simulink model "flightController"  (R2021b)
settings: Solver=ode3  StartTime=0  StopTime=TFinal  FixedStep=Ts  RelTol=1e-3  EnableMultiTasking=on
undefined symbols (not defined in the file): Controller, DiscIntNeverNeededParam, g, INDI, Ts, Vehicle
libraries: spsSecondOrderFilterLib x12, simulink x6
settings Model: Creator=The MathWorks, Inc.  LastModifiedBy=Tiga
settings SolverCC: AlgebraicLoopSolver=TrustRegion  MinimalZcImpactIntegration=on
settings DataIOCC: LimitDataPoints=on  SaveFormat=Array  ReturnWorkspaceOutputs=off
settings OptimizationCC: BlockReduction=off  DefaultParameterBehavior=Inlined  BufferReuse=off  PassReuseOutputArgsThreshold=0
settings DebuggingCC: AlgebraicLoopMsg=none  ParameterPrecisionLossMsg=none  ParameterTunabilityLossMsg=error  UnconnectedInputMsg=none  UnconnectedOutputMsg=none  UnconnectedLineMsg=none  BusObjectLabelMismatch=error  SFUnexpectedBacktrackingDiag=warning  SFNoUnconditionalDefaultTransitionDiag=warning  SFExecutionAtInitializationDiag=none  SFMachineParentedDataDiag=warning  ArithmeticOperatorsInVariantConditions=warning
settings HardwareCC: ProdBitPerPointer=32  ProdBitPerSizeT=32  ProdBitPerPtrDiffT=32  ProdLargestAtomicInteger=Long  ProdWordSize=32  ProdHWDeviceType=ARM Compatible->ARM 9
settings ModelReferenceCC: ModelReferenceNumInstancesAllowed=Single  PropagateSignalLabelsOutOfModel=off
settings SFSimCC: SimUseLocalCustomCode=off  CustomCodeUndefinedFunction=UseInterfaceOnly
settings RTWCC: GenerateReport=on  RTWUseLocalCustomCode=off  LaunchReport=on
settings CodeAppCC: ForceParamTrailComments=on  MaxIdLength=63  OperatorAnnotations=on  StateflowObjectComments=on  MATLABSourceComments=on
settings GRTTargetCC: TargetLangStandard=C89/C90 (ANSI)
settings ConfigComp: CovMetricSettings=dw  CovSaveCumulativeToWorkspaceVar=on  CovSaveSingleToWorkspaceVar=on  CovExternalEMLEnable=off  CovSFcnEnable=off

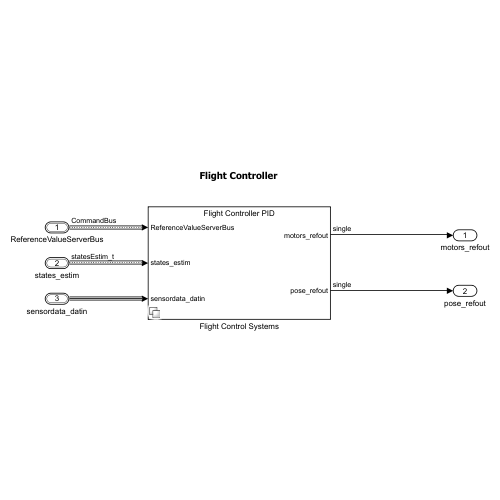
[thumbnail: Simulink's stored preview of the top-level diagram]
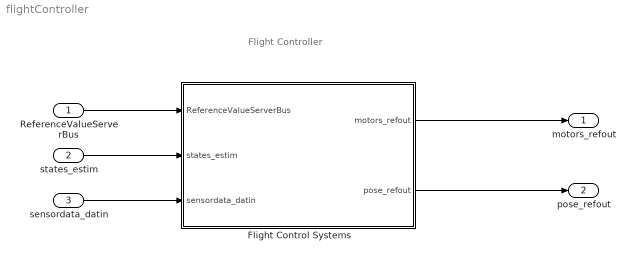
== system flightController ==
  note: Flight Controller
  ReferenceValueServerBus : Inport  OutDataTypeStr=Bus: CommandBus  BusOutputAsStruct=on
  states_estim : Inport  Port=2  OutDataTypeStr=Bus: statesEstim_t  BusOutputAsStruct=on
  sensordata_datin : Inport  Port=3  OutDataTypeStr=Bus: sensordata_t
  Flight Control Systems : Subsystem  Variant=on
  motors_refout : Outport  VectorParamsAs1DForOutWhenUnconnected=off
  pose_refout : Outport  Port=2  VectorParamsAs1DForOutWhenUnconnected=off
  wires:
  ReferenceValueServerBus/1 -> Flight Control Systems/1(ReferenceValueServerBus)
  states_estim/1 -> Flight Control Systems/2(states_estim)
  Flight Control Systems/2(pose_refout) -> pose_refout/1
  Flight Control Systems/1(motors_refout) -> motors_refout/1
  sensordata_datin/1 -> Flight Control Systems/3(sensordata_datin)

== system flightController/Flight Control Systems ==
  note: 1) Add Subsystem or Model blocks as valid variant choices.
      | 2) You cannot connect blocks at this level. At simulation, connectivity is automatically
      | determined, based on the active variant and port name matching.
  ReferenceValueServerBus : Inport
  states_estim : Inport  Port=2
  sensordata_datin : Inport  Port=3
  Flight Controller INDI : Subsystem  VariantControl=VSS_FCS_INDI
  Flight Controller PID : Subsystem  VariantControl=VSS_FCS_PID
  Flight Controller PID + INDI : Subsystem  VariantControl=VSS_FCS_PID_INDI
  motors_refout : Outport
  pose_refout : Outport  Port=2

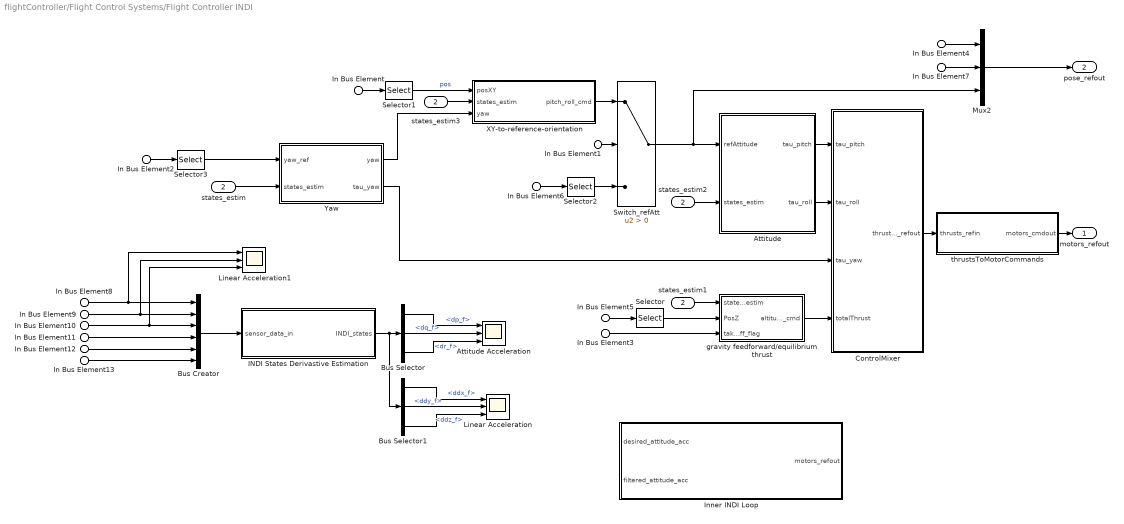
== system flightController/Flight Control Systems/Flight Controller INDI ==
  In Bus Element1 : Inport  PortName=ReferenceValueServerBus  Element=controlModePosVSOrient
  In Bus Element : Inport  PortName=ReferenceValueServerBus  Element=pos_ref
  In Bus Element4 : Inport  PortName=ReferenceValueServerBus  Element=pos_ref
  In Bus Element5 : Inport  PortName=ReferenceValueServerBus  Element=pos_ref
  In Bus Element2 : Inport  PortName=ReferenceValueServerBus  Element=orient_ref
  In Bus Element6 : Inport  PortName=ReferenceValueServerBus  Element=orient_ref
  In Bus Element7 : Inport  PortName=ReferenceValueServerBus  Element=orient_ref
  In Bus Element3 : Inport  PortName=ReferenceValueServerBus  Element=takeoff_flag
  states_estim : Inport  Port=2
  In Bus Element8 : Inport  Port=3  PortName=sensordata_datin  Element=ddx
  In Bus Element9 : Inport  Port=3  PortName=sensordata_datin  Element=ddy
  In Bus Element10 : Inport  Port=3  PortName=sensordata_datin  Element=ddz
  In Bus Element11 : Inport  Port=3  PortName=sensordata_datin  Element=p
  In Bus Element12 : Inport  Port=3  PortName=sensordata_datin  Element=q
  In Bus Element13 : Inport  Port=3  PortName=sensordata_datin  Element=r
  Attitude : Subsystem
  Attitude Acceleration : Scope  NumInputPorts=3
  Bus Creator : BusCreator  Inputs=6
  Bus Selector : BusSelector  OutputSignals=dp_f,dq_f,dr_f
  Bus Selector1 : BusSelector  OutputSignals=ddx_f,ddy_f,ddz_f
  ControlMixer : Subsystem
  INDI States Derivastive Estimation : Subsystem
  Inner INDI Loop : Subsystem
  Linear Acceleration : Scope  NumInputPorts=3
  Linear Acceleration1 : Scope  NumInputPorts=3
  Mux2 : Mux  Inputs=3
  Selector : Selector  InputPortWidth=3  IndexOptions=Index vector (dialog)  Indices=3  OutputSizes=1
  Selector1 : Selector  InputPortWidth=3  IndexOptions=Index vector (dialog)  Indices=[1 2]  OutputSizes=1
  Selector2 : Selector  InputPortWidth=3  IndexOptions=Index vector (dialog)  Indices=[2 3]  OutputSizes=1
  Selector3 : Selector  InputPortWidth=3  IndexOptions=Index vector (dialog)  Indices=1  OutputSizes=1
  Switch_refAtt : Switch  Criteria=u2 > Threshold
  XY-to-reference-orientation : Subsystem
  Yaw : Subsystem
  gravity feedforward/equilibrium thrust : Subsystem
  states_estim1 : InportShadow  Port=2
  states_estim2 : InportShadow  Port=2
  states_estim3 : InportShadow  Port=2
  thrustsToMotorCommands : Subsystem
  motors_refout : Outport  VectorParamsAs1DForOutWhenUnconnected=off
  pose_refout : Outport  Port=2  VectorParamsAs1DForOutWhenUnconnected=off
  wires:
  thrustsToMotorCommands/1(motors_cmdout) -> motors_refout/1
  In Bus Element1/1 -> Switch_refAtt/2
  XY-to-reference-orientation/1(pitch_roll_cmd) -> Switch_refAtt/1
  In Bus Element2/1 -> Selector3/1
  In Bus Element/1 -> Selector1/1
  Selector3/1 -> Yaw/1(yaw_ref)
  Selector1/1 -> XY-to-reference-orientation/1(posXY)  "pos"
  ControlMixer/1(thrusts_refout) -> thrustsToMotorCommands/1(thrusts_refin)
  In Bus Element3/1 -> gravity feedforward/equilibrium thrust/3(takeoff_flag)
  states_estim/1 -> Yaw/2(states_estim)
  Switch_refAtt/1 -> Attitude/1(refAttitude), Mux2/3
  Yaw/1(yaw) -> XY-to-reference-orientation/3(yaw)
  gravity feedforward/equilibrium thrust/1(altitude_cmd) -> ControlMixer/4(totalThrust)
  Mux2/1 -> pose_refout/1
  Attitude/1(tau_pitch) -> ControlMixer/1(tau_pitch)
  Attitude/2(tau_roll) -> ControlMixer/2(tau_roll)
  Yaw/2(tau_yaw) -> ControlMixer/3(tau_yaw)
  states_estim1/1 -> gravity feedforward/equilibrium thrust/1(states_estim)
  states_estim2/1 -> Attitude/2(states_estim)
  states_estim3/1 -> XY-to-reference-orientation/2(states_estim)
  In Bus Element4/1 -> Mux2/1
  Selector/1 -> gravity feedforward/equilibrium thrust/2(PosZ)
  In Bus Element5/1 -> Selector/1
  In Bus Element6/1 -> Selector2/1
  Selector2/1 -> Switch_refAtt/3
  In Bus Element7/1 -> Mux2/2
  INDI States Derivastive Estimation/1(INDI_states) -> Bus Selector1/1, Bus Selector/1
  Bus Selector/1 -> Attitude Acceleration/1  "<dp_f>"
  Bus Selector/2 -> Attitude Acceleration/2  "<dq_f>"
  Bus Selector/3 -> Attitude Acceleration/3  "<dr_f>"
  In Bus Element8/1 -> Bus Creator/1, Linear Acceleration1/1
  In Bus Element9/1 -> Bus Creator/2, Linear Acceleration1/2
  In Bus Element10/1 -> Bus Creator/3, Linear Acceleration1/3
  In Bus Element11/1 -> Bus Creator/4
  In Bus Element13/1 -> Bus Creator/6
  In Bus Element12/1 -> Bus Creator/5
  Bus Creator/1 -> INDI States Derivastive Estimation/1(sensor_data_in)
  Bus Selector1/1 -> Linear Acceleration/1  "<ddx_f>"
  Bus Selector1/2 -> Linear Acceleration/2  "<ddy_f>"
  Bus Selector1/3 -> Linear Acceleration/3  "<ddz_f>"

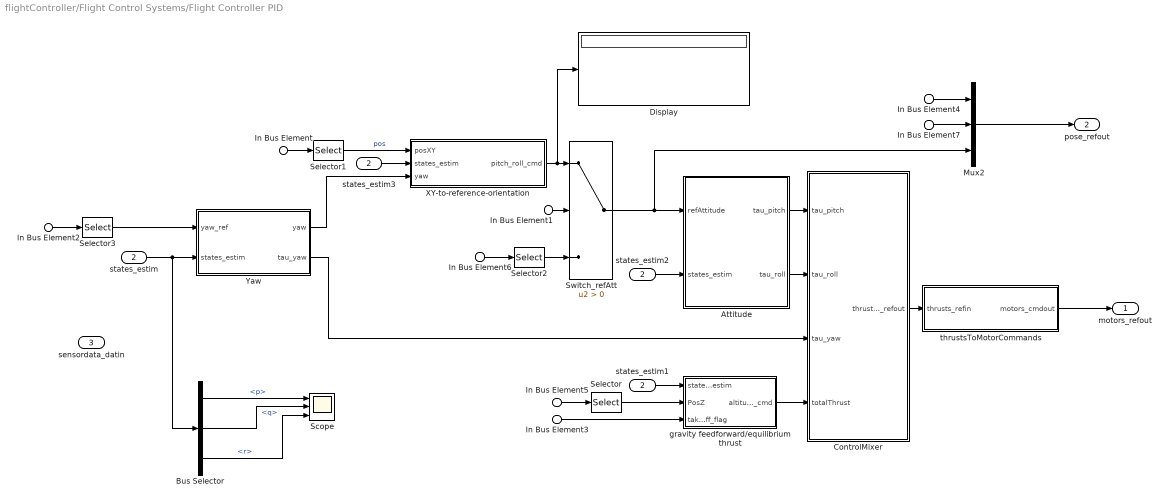
== system flightController/Flight Control Systems/Flight Controller PID ==
  In Bus Element1 : Inport  PortName=ReferenceValueServerBus  Element=controlModePosVSOrient
  In Bus Element : Inport  PortName=ReferenceValueServerBus  Element=pos_ref
  In Bus Element4 : Inport  PortName=ReferenceValueServerBus  Element=pos_ref
  In Bus Element5 : Inport  PortName=ReferenceValueServerBus  Element=pos_ref
  In Bus Element2 : Inport  PortName=ReferenceValueServerBus  Element=orient_ref
  In Bus Element6 : Inport  PortName=ReferenceValueServerBus  Element=orient_ref
  In Bus Element7 : Inport  PortName=ReferenceValueServerBus  Element=orient_ref
  In Bus Element3 : Inport  PortName=ReferenceValueServerBus  Element=takeoff_flag
  states_estim : Inport  Port=2
  sensordata_datin : Inport  Port=3
  Attitude : Subsystem
  Bus Selector : BusSelector  OutputSignals=p,q,r
  ControlMixer : Subsystem
  Display : Display
  Mux2 : Mux  Inputs=3
  Scope : Scope  NumInputPorts=3
  Selector : Selector  InputPortWidth=3  IndexOptions=Index vector (dialog)  Indices=3  OutputSizes=1
  Selector1 : Selector  InputPortWidth=3  IndexOptions=Index vector (dialog)  Indices=[1 2]  OutputSizes=1
  Selector2 : Selector  InputPortWidth=3  IndexOptions=Index vector (dialog)  Indices=[2 3]  OutputSizes=1
  Selector3 : Selector  InputPortWidth=3  IndexOptions=Index vector (dialog)  Indices=1  OutputSizes=1
  Switch_refAtt : Switch  Criteria=u2 > Threshold
  XY-to-reference-orientation : Subsystem
  Yaw : Subsystem
  gravity feedforward/equilibrium thrust : Subsystem
  states_estim1 : InportShadow  Port=2
  states_estim2 : InportShadow  Port=2
  states_estim3 : InportShadow  Port=2
  thrustsToMotorCommands : Subsystem
  motors_refout : Outport  VectorParamsAs1DForOutWhenUnconnected=off
  pose_refout : Outport  Port=2  VectorParamsAs1DForOutWhenUnconnected=off
  wires:
  thrustsToMotorCommands/1(motors_cmdout) -> motors_refout/1
  In Bus Element1/1 -> Switch_refAtt/2
  XY-to-reference-orientation/1(pitch_roll_cmd) -> Display/1, Switch_refAtt/1
  In Bus Element2/1 -> Selector3/1
  In Bus Element/1 -> Selector1/1
  Selector3/1 -> Yaw/1(yaw_ref)
  Selector1/1 -> XY-to-reference-orientation/1(posXY)  "pos"
  ControlMixer/1(thrusts_refout) -> thrustsToMotorCommands/1(thrusts_refin)
  In Bus Element3/1 -> gravity feedforward/equilibrium thrust/3(takeoff_flag)
  states_estim/1 -> Bus Selector/1, Yaw/2(states_estim)
  Switch_refAtt/1 -> Attitude/1(refAttitude), Mux2/3
  Yaw/1(yaw) -> XY-to-reference-orientation/3(yaw)
  gravity feedforward/equilibrium thrust/1(altitude_cmd) -> ControlMixer/4(totalThrust)
  Mux2/1 -> pose_refout/1
  Attitude/1(tau_pitch) -> ControlMixer/1(tau_pitch)
  Attitude/2(tau_roll) -> ControlMixer/2(tau_roll)
  Yaw/2(tau_yaw) -> ControlMixer/3(tau_yaw)
  states_estim1/1 -> gravity feedforward/equilibrium thrust/1(states_estim)
  states_estim2/1 -> Attitude/2(states_estim)
  states_estim3/1 -> XY-to-reference-orientation/2(states_estim)
  In Bus Element4/1 -> Mux2/1
  Selector/1 -> gravity feedforward/equilibrium thrust/2(PosZ)
  In Bus Element5/1 -> Selector/1
  In Bus Element6/1 -> Selector2/1
  Selector2/1 -> Switch_refAtt/3
  In Bus Element7/1 -> Mux2/2
  Bus Selector/1 -> Scope/1  "<p>"
  Bus Selector/2 -> Scope/2  "<q>"
  Bus Selector/3 -> Scope/3  "<r>"

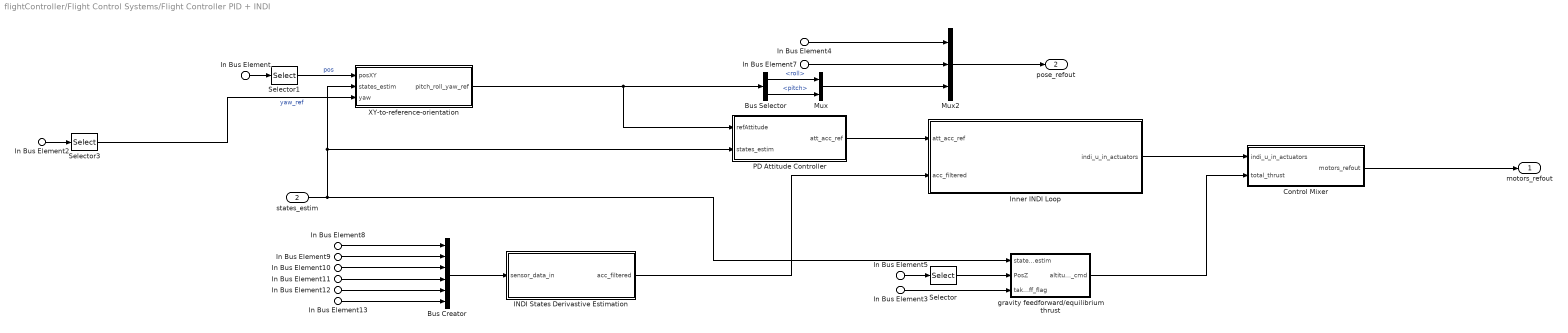
== system flightController/Flight Control Systems/Flight Controller PID + INDI ==
  In Bus Element : Inport  PortName=ReferenceValueServerBus  Element=pos_ref
  In Bus Element4 : Inport  PortName=ReferenceValueServerBus  Element=pos_ref
  In Bus Element5 : Inport  PortName=ReferenceValueServerBus  Element=pos_ref
  In Bus Element2 : Inport  PortName=ReferenceValueServerBus  Element=orient_ref
  In Bus Element7 : Inport  PortName=ReferenceValueServerBus  Element=orient_ref
  In Bus Element3 : Inport  PortName=ReferenceValueServerBus  Element=takeoff_flag
  states_estim : Inport  Port=2
  In Bus Element8 : Inport  Port=3  PortName=sensordata_datin  Element=ddx
  In Bus Element9 : Inport  Port=3  PortName=sensordata_datin  Element=ddy
  In Bus Element10 : Inport  Port=3  PortName=sensordata_datin  Element=ddz
  In Bus Element11 : Inport  Port=3  PortName=sensordata_datin  Element=p
  In Bus Element12 : Inport  Port=3  PortName=sensordata_datin  Element=q
  In Bus Element13 : Inport  Port=3  PortName=sensordata_datin  Element=r
  Bus Creator : BusCreator  Inputs=6
  Bus Selector : BusSelector  OutputSignals=roll,pitch
  Control Mixer : Subsystem
  INDI States Derivastive Estimation : Subsystem
  Inner INDI Loop : Subsystem
  Mux : Mux  Inputs=2
  Mux2 : Mux  Inputs=3
  PD Attitude Controller : Subsystem
  Selector : Selector  InputPortWidth=3  IndexOptions=Index vector (dialog)  Indices=3  OutputSizes=1
  Selector1 : Selector  InputPortWidth=3  IndexOptions=Index vector (dialog)  Indices=[1 2]  OutputSizes=1
  Selector3 : Selector  InputPortWidth=3  IndexOptions=Index vector (dialog)  Indices=1  OutputSizes=1
  XY-to-reference-orientation : Subsystem
  gravity feedforward/equilibrium thrust : Subsystem
  motors_refout : Outport  OutDataTypeStr=single  VectorParamsAs1DForOutWhenUnconnected=off
  pose_refout : Outport  Port=2  VectorParamsAs1DForOutWhenUnconnected=off
  wires:
  XY-to-reference-orientation/1(pitch_roll_yaw_ref) -> Bus Selector/1, PD Attitude Controller/1(refAttitude)
  In Bus Element2/1 -> Selector3/1
  In Bus Element/1 -> Selector1/1
  Selector1/1 -> XY-to-reference-orientation/1(posXY)  "pos"
  In Bus Element3/1 -> gravity feedforward/equilibrium thrust/3(takeoff_flag)
  gravity feedforward/equilibrium thrust/1(altitude_cmd) -> Control Mixer/2(total_thrust)
  Mux2/1 -> pose_refout/1
  states_estim/1 -> gravity feedforward/equilibrium thrust/1(states_estim), PD Attitude Controller/2(states_estim), XY-to-reference-orientation/2(states_estim)
  In Bus Element4/1 -> Mux2/1
  Selector/1 -> gravity feedforward/equilibrium thrust/2(PosZ)
  In Bus Element5/1 -> Selector/1
  In Bus Element7/1 -> Mux2/2
  INDI States Derivastive Estimation/1(acc_filtered) -> Inner INDI Loop/2(acc_filtered)
  In Bus Element8/1 -> Bus Creator/1
  In Bus Element9/1 -> Bus Creator/2
  In Bus Element10/1 -> Bus Creator/3
  In Bus Element11/1 -> Bus Creator/4
  In Bus Element13/1 -> Bus Creator/6
  In Bus Element12/1 -> Bus Creator/5
  Bus Creator/1 -> INDI States Derivastive Estimation/1(sensor_data_in)
  PD Attitude Controller/1(att_acc_ref) -> Inner INDI Loop/1(att_acc_ref)
  Selector3/1 -> XY-to-reference-orientation/3(yaw)  "yaw_ref"
  Inner INDI Loop/1(indi_u_in_actuators) -> Control Mixer/1(indi_u_in_actuators)
  Bus Selector/1 -> Mux/1  "<roll>"
  Bus Selector/2 -> Mux/2  "<pitch>"
  Mux/1 -> Mux2/3
  Control Mixer/1(motors_refout) -> motors_refout/1

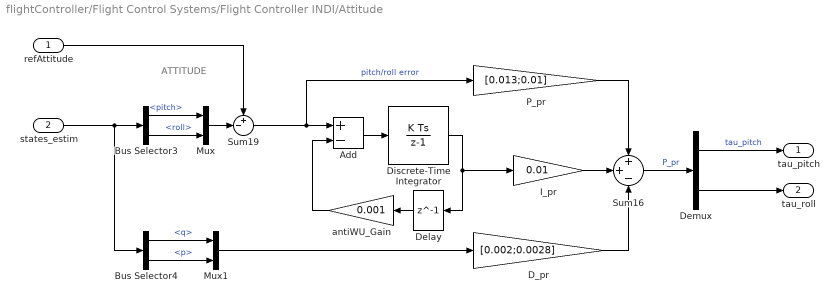
== system flightController/Flight Control Systems/Flight Controller INDI/Attitude ==
  note: ATTITUDE
  refAttitude : Inport
  states_estim : Inport  Port=2
  Add : Sum  Inputs=+-
  Bus Selector3 : BusSelector  OutputSignals=pitch,roll
  Bus Selector4 : BusSelector  OutputSignals=q,p
  D_pr : Gain  Gain=[0.002;0.0028]
  Delay : Delay  DelayLength=1  InitialCondition=0
  Demux : Demux  Outputs=2
  Discrete-Time Integrator : DiscreteIntegrator  SampleTime=Ts  LimitOutput=on  UpperSaturationLimit=2  LowerSaturationLimit=-2  ICPrevOutput=DiscIntNeverNeededParam  ICPrevScaledInput=DiscIntNeverNeededParam
  I_pr : Gain  Gain=0.01
  Mux : Mux  Inputs=2
  Mux1 : Mux  Inputs=2
  P_pr : Gain  Gain=[0.013;0.01]
  Sum16 : Sum  Inputs=++-  AccumDataTypeStr=single  OutDataTypeStr=single  SaturateOnIntegerOverflow=on
  Sum19 : Sum  Inputs=+-|
  antiWU_Gain : Gain  Gain=0.001
  tau_pitch : Outport  VectorParamsAs1DForOutWhenUnconnected=off
  tau_roll : Outport  Port=2  VectorParamsAs1DForOutWhenUnconnected=off
  wires:
  Sum16/1 -> Demux/1  "P_pr"
  antiWU_Gain/1 -> Add/2
  Add/1 -> Discrete-Time Integrator/1
  Bus Selector3/1 -> Mux/1  "<pitch>"
  Bus Selector4/1 -> Mux1/1  "<q>"
  P_pr/1 -> Sum16/1
  I_pr/1 -> Sum16/2
  Sum19/1 -> Add/1, P_pr/1  "pitch/roll error"
  Discrete-Time Integrator/1 -> Delay/1, I_pr/1
  Delay/1 -> antiWU_Gain/1
  Demux/1 -> tau_pitch/1  "tau_pitch"
  Demux/2 -> tau_roll/1
  D_pr/1 -> Sum16/3
  states_estim/1 -> Bus Selector3/1, Bus Selector4/1
  refAttitude/1 -> Sum19/1
  Mux/1 -> Sum19/2
  Bus Selector3/2 -> Mux/2  "<roll>"
  Mux1/1 -> D_pr/1
  Bus Selector4/2 -> Mux1/2  "<p>"

== system flightController/Flight Control Systems/Flight Controller INDI/ControlMixer ==
  tau_pitch : Inport
  tau_roll : Inport  Port=2
  tau_yaw : Inport  Port=3
  totalThrust : Inport  Port=4
  Mux2 : Mux
  Product : Product  Multiplication=Matrix(*)  RndMeth=Zero
  TorqueTotalThrustToThrustPerMotor : Constant  Value=Controller.Q2Ts  OutDataTypeStr=single
  thrusts_refout : Outport  VectorParamsAs1DForOutWhenUnconnected=off
  wires:
  Product/1 -> thrusts_refout/1
  tau_roll/1 -> Mux2/4
  tau_pitch/1 -> Mux2/3
  tau_yaw/1 -> Mux2/2
  totalThrust/1 -> Mux2/1
  TorqueTotalThrustToThrustPerMotor/1 -> Product/1
  Mux2/1 -> Product/2

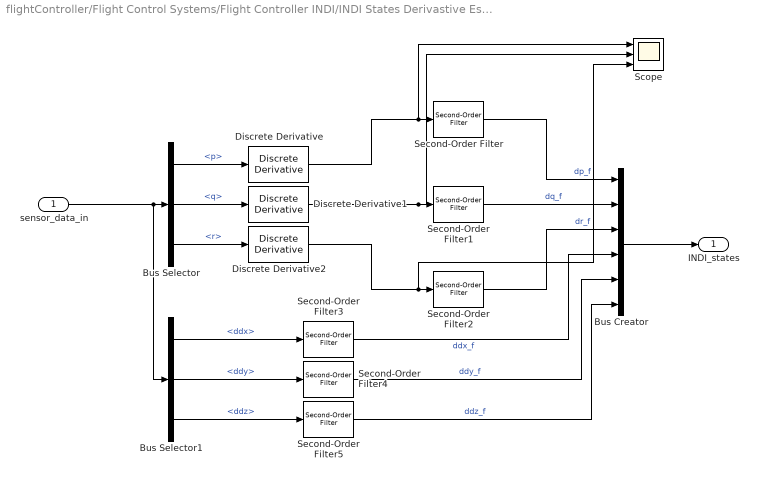
== system flightController/Flight Control Systems/Flight Controller INDI/INDI States Derivastive Estimation ==
  sensor_data_in : Inport
  Bus Creator : BusCreator  Inputs=6
  Bus Selector : BusSelector  OutputSignals=p,q,r
  Bus Selector1 : BusSelector  OutputSignals=ddx,ddy,ddz
  Discrete Derivative : simulink/Discrete/Discrete Derivative  gainval=1.0  ICPrevScaledInput=0.0  OutMin=[]  OutMax=[]  OutDataType=fixdt(1, 16)  OutScaling=2^-10  DoSatur=off
  Discrete Derivative1 : simulink/Discrete/Discrete Derivative  gainval=1.0  ICPrevScaledInput=0.0  OutMin=[]  OutMax=[]  OutDataType=fixdt(1, 16)  OutScaling=2^-10  DoSatur=off
  Discrete Derivative2 : simulink/Discrete/Discrete Derivative  gainval=1.0  ICPrevScaledInput=0.0  OutMin=[]  OutMax=[]  OutDataType=fixdt(1, 16)  OutScaling=2^-10  DoSatur=off
  Scope : Scope  NumInputPorts=3
  Second-Order Filter{,1..5} (6 alike) : spsSecondOrderFilterLib/Second-Order Filter  FilterType=Lowpass  Fo=7.9577  Zeta=0.55  Ts=0.005  Initialize=on  Vac_Init="[0,  0,  60]"  Vdc_Init=0  PlotResponse=off  FreqRange=[0, 500, 1]
      settings: SourceProductBaseCode=PS
  INDI_states : Outport
  wires:
  sensor_data_in/1 -> Bus Selector1/1, Bus Selector/1
  Second-Order Filter/1 -> Bus Creator/1  "dp_f"
  Second-Order Filter1/1 -> Bus Creator/2  "dq_f"
  Second-Order Filter2/1 -> Bus Creator/3  "dr_f"
  Bus Creator/1 -> INDI_states/1
  Bus Selector/1 -> Discrete Derivative/1  "<p>"
  Bus Selector/2 -> Discrete Derivative1/1  "<q>"
  Bus Selector/3 -> Discrete Derivative2/1  "<r>"
  Discrete Derivative/1 -> Scope/1, Second-Order Filter/1
  Discrete Derivative1/1 -> Scope/2, Second-Order Filter1/1
  Discrete Derivative2/1 -> Scope/3, Second-Order Filter2/1
  Bus Selector1/1 -> Second-Order Filter3/1  "<ddx>"
  Bus Selector1/2 -> Second-Order Filter4/1  "<ddy>"
  Bus Selector1/3 -> Second-Order Filter5/1  "<ddz>"
  Second-Order Filter3/1 -> Bus Creator/4  "ddx_f"
  Second-Order Filter4/1 -> Bus Creator/5  "ddy_f"
  Second-Order Filter5/1 -> Bus Creator/6  "ddz_f"

== system flightController/Flight Control Systems/Flight Controller INDI/Inner INDI Loop ==
  desired_attitude_acc : Inport
  filtered_attitude_acc : Inport  Port=2
  Add : Sum
  Add1 : Sum
  G2 : Gain  Gain=INDI.G2
  Plus : Sum  Inputs=+-
  Unit Delay : UnitDelay  SampleTime=-1  HasFrameUpgradeWarning=on
  Unit Delay1 : UnitDelay  SampleTime=-1  HasFrameUpgradeWarning=on
  inv(G1+G2) : Gain  Gain=INDI.G1G2_inv  Multiplication=Matrix(K*u)
  motor-speed to motor-cmd : Subsystem
  motors_refout : Outport
  wires:
  desired_attitude_acc/1 -> Plus/1
  filtered_attitude_acc/1 -> Plus/2
  Plus/1 -> Add/1  "attitude_acc_error"
  Add/1 -> inv(G1+G2)/1
  Unit Delay/1 -> G2/1
  G2/1 -> Add/2
  inv(G1+G2)/1 -> Add1/1, Unit Delay/1  "delta_motor_w"
  Unit Delay1/1 -> Add1/2  "motor_w_f"
  Add1/1 -> Unit Delay1/1, motor-speed to motor-cmd/1(motor_w_c)  "motor_w_c"
  motor-speed to motor-cmd/1(motors_refout) -> motors_refout/1

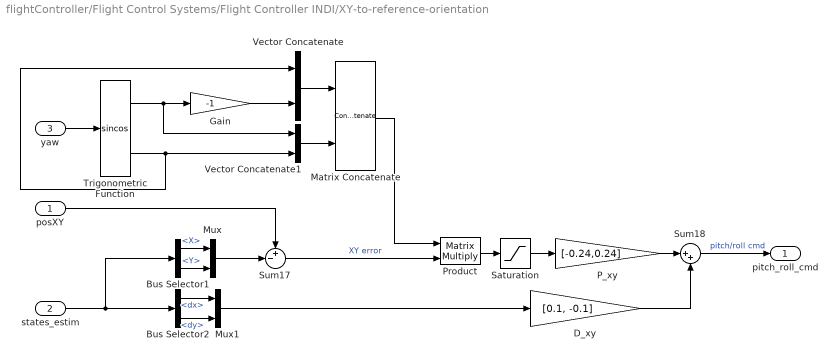
== system flightController/Flight Control Systems/Flight Controller INDI/XY-to-reference-orientation ==
  posXY : Inport
  states_estim : Inport  Port=2
  yaw : Inport  Port=3
  Bus Selector1 : BusSelector  OutputSignals=X,Y
  Bus Selector2 : BusSelector  OutputSignals=dx,dy
  D_xy : Gain  Gain=[0.1, -0.1]  ParamDataTypeStr=single  OutDataTypeStr=single  SaturateOnIntegerOverflow=on
  Gain : Gain  Gain=-1
  Matrix Concatenate : Concatenate  Mode=Multidimensional array  ConcatenateDimension=2
  Mux : Mux  Inputs=2
  Mux1 : Mux  Inputs=2
  P_xy : Gain  Gain=[-0.24,0.24]  ParamDataTypeStr=single  OutDataTypeStr=single  SaturateOnIntegerOverflow=on
  Product : Product  Multiplication=Matrix(*)  OutDataTypeStr=single  RndMeth=Zero
  Saturation : Saturate  UpperLimit=3  LowerLimit=-3  OutDataTypeStr=single
  Sum17 : Sum  Inputs=+-|  AccumDataTypeStr=single
  Sum18 : Sum  Inputs=|++  AccumDataTypeStr=single  OutDataTypeStr=single  SaturateOnIntegerOverflow=on
  Trigonometric Function : Trigonometry  Operator=sincos
  Vector Concatenate : Concatenate
  Vector Concatenate1 : Concatenate
  pitch_roll_cmd : Outport  VectorParamsAs1DForOutWhenUnconnected=off
  wires:
  yaw/1 -> Trigonometric Function/1
  Saturation/1 -> P_xy/1
  P_xy/1 -> Sum18/1
  Sum17/1 -> Product/2  "XY error"
  posXY/1 -> Sum17/1
  Bus Selector2/1 -> Mux1/1  "<dx>"
  states_estim/1 -> Bus Selector1/1, Bus Selector2/1
  Sum18/1 -> pitch_roll_cmd/1  "pitch/roll cmd"
  D_xy/1 -> Sum18/2
  Bus Selector1/1 -> Mux/1  "<X>"
  Product/1 -> Saturation/1
  Trigonometric Function/1 -> Gain/1, Vector Concatenate1/1
  Trigonometric Function/2 -> Vector Concatenate1/2, Vector Concatenate/1
  Gain/1 -> Vector Concatenate/2
  Vector Concatenate/1 -> Matrix Concatenate/1
  Vector Concatenate1/1 -> Matrix Concatenate/2
  Matrix Concatenate/1 -> Product/1
  Bus Selector1/2 -> Mux/2  "<Y>"
  Mux/1 -> Sum17/2
  Mux1/1 -> D_xy/1
  Bus Selector2/2 -> Mux1/2  "<dy>"

== system flightController/Flight Control Systems/Flight Controller INDI/Yaw ==
  yaw_ref : Inport
  states_estim : Inport  Port=2
  Bus Selector5 : BusSelector  OutputSignals=yaw,r
  D_yaw : Gain  Gain=0.3*0.004
  P_yaw : Gain  Gain=0.004  ParamDataTypeStr=single  OutDataTypeStr=single
  Sum1 : Sum  Inputs=+-|  AccumDataTypeStr=single  OutDataTypeStr=single  SaturateOnIntegerOverflow=on
  Sum2 : Sum  Inputs=|+-
  yaw : Outport  VectorParamsAs1DForOutWhenUnconnected=off
  tau_yaw : Outport  Port=2  VectorParamsAs1DForOutWhenUnconnected=off
  wires:
  D_yaw/1 -> Sum2/2
  P_yaw/1 -> Sum2/1
  Bus Selector5/2 -> D_yaw/1  "<r>"
  Sum1/1 -> P_yaw/1
  states_estim/1 -> Bus Selector5/1
  Sum2/1 -> tau_yaw/1
  Bus Selector5/1 -> yaw/1, Sum1/2  "<yaw>"
  yaw_ref/1 -> Sum1/1

== system flightController/Flight Control Systems/Flight Controller INDI/gravity feedforward//equilibrium thrust ==
  note: ALTITUDE
  states_estim : Inport
  PosZ : Inport  Port=2
  takeoff_flag : Inport  Port=3
  Bus Selector6 : BusSelector  OutputSignals=Z,dz
  D_z : Gain  Gain=0.3  ParamDataTypeStr=single  OutDataTypeStr=single  SaturateOnIntegerOverflow=on
  P_z : Gain  Gain=0.8  ParamDataTypeStr=single  OutDataTypeStr=single  SaturateOnIntegerOverflow=on
  SaturationThrust : Saturate  UpperLimit=4*Controller.totalThrustMaxRelative*Controller.motorsThrustPerMotorMax  LowerLimit=-4*Controller.totalThrustMaxRelative*Controller.motorsThrustPerMotorMax  OutDataTypeStr=single
  Sum15 : Sum  Inputs=|+-  AccumDataTypeStr=single  OutDataTypeStr=single  SaturateOnIntegerOverflow=on
  Sum3 : Sum  Inputs=+-|  AccumDataTypeStr=single  OutDataTypeStr=single  SaturateOnIntegerOverflow=on
  Sum4 : Sum  Inputs=++|  AccumDataTypeStr=single  OutDataTypeStr=single  SaturateOnIntegerOverflow=on
  TakeoffOrControl_Switch : Switch  Criteria=u2 > Threshold
  takeoff_gain : Gain  Gain=Controller.takeoffGain  ParamDataTypeStr=single  OutDataTypeStr=single  SaturateOnIntegerOverflow=on
  w0 : Constant  Value=-g*Vehicle.Airframe.mass  OutDataTypeStr=single  SampleTime=Ts
  altitude_cmd : Outport  VectorParamsAs1DForOutWhenUnconnected=off
  wires:
  Sum3/1 -> P_z/1  "errZ"
  TakeoffOrControl_Switch/1 -> Sum4/2
  Bus Selector6/1 -> Sum3/2  "<Z>"
  Bus Selector6/2 -> D_z/1  "<dz>"
  w0/1 -> Sum4/1, takeoff_gain/1
  D_z/1 -> Sum15/2  "dz"
  takeoff_gain/1 -> TakeoffOrControl_Switch/1
  takeoff_flag/1 -> TakeoffOrControl_Switch/2
  PosZ/1 -> Sum3/1
  P_z/1 -> Sum15/1
  Sum15/1 -> TakeoffOrControl_Switch/3
  Sum4/1 -> SaturationThrust/1
  SaturationThrust/1 -> altitude_cmd/1
  states_estim/1 -> Bus Selector6/1

== system flightController/Flight Control Systems/Flight Controller INDI/thrustsToMotorCommands ==
  thrusts_refin : Inport
  MotorDirections : Gain  Gain=[1 -1 1 -1]
  Saturation5 : Saturate  UpperLimit=Vehicle.Motor.maxLimit  LowerLimit=Vehicle.Motor.minLimit
  ThrustToMotorCommand : Gain  Gain=-Vehicle.Motor.thrustToMotorCommand
  motors_cmdout : Outport  VectorParamsAs1DForOutWhenUnconnected=off
  wires:
  Saturation5/1 -> MotorDirections/1
  MotorDirections/1 -> motors_cmdout/1
  ThrustToMotorCommand/1 -> Saturation5/1
  thrusts_refin/1 -> ThrustToMotorCommand/1

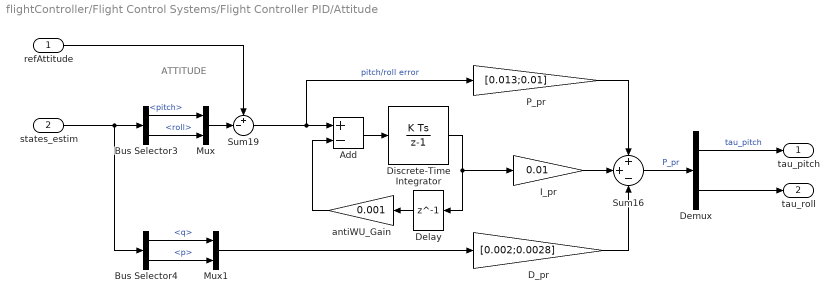
== system flightController/Flight Control Systems/Flight Controller PID/Attitude ==
  note: ATTITUDE
  refAttitude : Inport
  states_estim : Inport  Port=2
  Add : Sum  Inputs=+-
  Bus Selector3 : BusSelector  OutputSignals=pitch,roll
  Bus Selector4 : BusSelector  OutputSignals=q,p
  D_pr : Gain  Gain=[0.002;0.0028]
  Delay : Delay  DelayLength=1  InitialCondition=0
  Demux : Demux  Outputs=2
  Discrete-Time Integrator : DiscreteIntegrator  SampleTime=Ts  LimitOutput=on  UpperSaturationLimit=2  LowerSaturationLimit=-2  ICPrevOutput=DiscIntNeverNeededParam  ICPrevScaledInput=DiscIntNeverNeededParam
  I_pr : Gain  Gain=0.01
  Mux : Mux  Inputs=2
  Mux1 : Mux  Inputs=2
  P_pr : Gain  Gain=[0.013;0.01]
  Sum16 : Sum  Inputs=++-  AccumDataTypeStr=single  OutDataTypeStr=single  SaturateOnIntegerOverflow=on
  Sum19 : Sum  Inputs=+-|
  antiWU_Gain : Gain  Gain=0.001
  tau_pitch : Outport  VectorParamsAs1DForOutWhenUnconnected=off
  tau_roll : Outport  Port=2  VectorParamsAs1DForOutWhenUnconnected=off
  wires:
  Sum16/1 -> Demux/1  "P_pr"
  antiWU_Gain/1 -> Add/2
  Add/1 -> Discrete-Time Integrator/1
  Bus Selector3/1 -> Mux/1  "<pitch>"
  Bus Selector4/1 -> Mux1/1  "<q>"
  P_pr/1 -> Sum16/1
  I_pr/1 -> Sum16/2
  Sum19/1 -> Add/1, P_pr/1  "pitch/roll error"
  Discrete-Time Integrator/1 -> Delay/1, I_pr/1
  Delay/1 -> antiWU_Gain/1
  Demux/1 -> tau_pitch/1  "tau_pitch"
  Demux/2 -> tau_roll/1
  D_pr/1 -> Sum16/3
  states_estim/1 -> Bus Selector3/1, Bus Selector4/1
  refAttitude/1 -> Sum19/1
  Mux/1 -> Sum19/2
  Bus Selector3/2 -> Mux/2  "<roll>"
  Mux1/1 -> D_pr/1
  Bus Selector4/2 -> Mux1/2  "<p>"

== system flightController/Flight Control Systems/Flight Controller PID/ControlMixer ==
  tau_pitch : Inport
  tau_roll : Inport  Port=2
  tau_yaw : Inport  Port=3
  totalThrust : Inport  Port=4
  Display : Display
  Mux2 : Mux
  Product : Product  Multiplication=Matrix(*)  RndMeth=Zero
  ThrustToMotorCommand : Gain  Gain=-Vehicle.Motor.thrustToMotorCommand
  TorqueTotalThrustToThrustPerMotor : Constant  Value=Controller.Q2Ts  OutDataTypeStr=single
  total thrust2cmd require for z pos : Display
  thrusts_refout : Outport  VectorParamsAs1DForOutWhenUnconnected=off
  wires:
  Product/1 -> thrusts_refout/1
  tau_roll/1 -> Mux2/4
  tau_pitch/1 -> Mux2/3
  tau_yaw/1 -> Mux2/2
  totalThrust/1 -> Display/1, ThrustToMotorCommand/1, Mux2/1
  TorqueTotalThrustToThrustPerMotor/1 -> Product/1
  Mux2/1 -> Product/2
  ThrustToMotorCommand/1 -> total thrust2cmd require for z pos/1

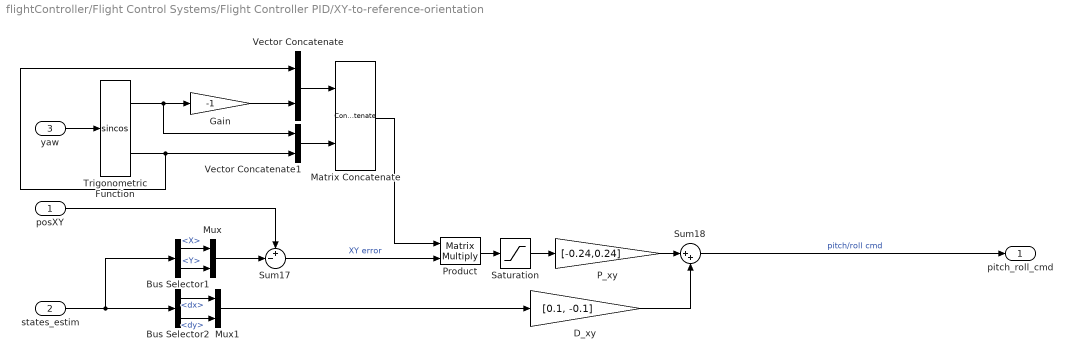
== system flightController/Flight Control Systems/Flight Controller PID/XY-to-reference-orientation ==
  posXY : Inport
  states_estim : Inport  Port=2
  yaw : Inport  Port=3
  Bus Selector1 : BusSelector  OutputSignals=X,Y
  Bus Selector2 : BusSelector  OutputSignals=dx,dy
  D_xy : Gain  Gain=[0.1, -0.1]  ParamDataTypeStr=single  OutDataTypeStr=single  SaturateOnIntegerOverflow=on
  Gain : Gain  Gain=-1
  Matrix Concatenate : Concatenate  Mode=Multidimensional array  ConcatenateDimension=2
  Mux : Mux  Inputs=2
  Mux1 : Mux  Inputs=2
  P_xy : Gain  Gain=[-0.24,0.24]  ParamDataTypeStr=single  OutDataTypeStr=single  SaturateOnIntegerOverflow=on
  Product : Product  Multiplication=Matrix(*)  OutDataTypeStr=single  RndMeth=Zero
  Saturation : Saturate  UpperLimit=3  LowerLimit=-3  OutDataTypeStr=single
  Sum17 : Sum  Inputs=+-|  AccumDataTypeStr=single
  Sum18 : Sum  Inputs=|++  AccumDataTypeStr=single  OutDataTypeStr=single  SaturateOnIntegerOverflow=on
  Trigonometric Function : Trigonometry  Operator=sincos
  Vector Concatenate : Concatenate
  Vector Concatenate1 : Concatenate
  pitch_roll_cmd : Outport  VectorParamsAs1DForOutWhenUnconnected=off
  wires:
  yaw/1 -> Trigonometric Function/1
  Saturation/1 -> P_xy/1
  P_xy/1 -> Sum18/1
  Sum17/1 -> Product/2  "XY error"
  posXY/1 -> Sum17/1
  Bus Selector2/1 -> Mux1/1  "<dx>"
  states_estim/1 -> Bus Selector1/1, Bus Selector2/1
  Sum18/1 -> pitch_roll_cmd/1  "pitch/roll cmd"
  D_xy/1 -> Sum18/2
  Bus Selector1/1 -> Mux/1  "<X>"
  Product/1 -> Saturation/1
  Trigonometric Function/1 -> Gain/1, Vector Concatenate1/1
  Trigonometric Function/2 -> Vector Concatenate1/2, Vector Concatenate/1
  Gain/1 -> Vector Concatenate/2
  Vector Concatenate/1 -> Matrix Concatenate/1
  Vector Concatenate1/1 -> Matrix Concatenate/2
  Matrix Concatenate/1 -> Product/1
  Bus Selector1/2 -> Mux/2  "<Y>"
  Mux/1 -> Sum17/2
  Mux1/1 -> D_xy/1
  Bus Selector2/2 -> Mux1/2  "<dy>"

== system flightController/Flight Control Systems/Flight Controller PID/Yaw ==
  yaw_ref : Inport
  states_estim : Inport  Port=2
  Bus Selector5 : BusSelector  OutputSignals=yaw,r
  D_yaw : Gain  Gain=0.3*0.004
  P_yaw : Gain  Gain=0.004  ParamDataTypeStr=single  OutDataTypeStr=single
  Sum1 : Sum  Inputs=+-|  AccumDataTypeStr=single  OutDataTypeStr=single  SaturateOnIntegerOverflow=on
  Sum2 : Sum  Inputs=|+-
  yaw : Outport  VectorParamsAs1DForOutWhenUnconnected=off
  tau_yaw : Outport  Port=2  VectorParamsAs1DForOutWhenUnconnected=off
  wires:
  D_yaw/1 -> Sum2/2
  P_yaw/1 -> Sum2/1
  Bus Selector5/2 -> D_yaw/1  "<r>"
  Sum1/1 -> P_yaw/1
  states_estim/1 -> Bus Selector5/1
  Sum2/1 -> tau_yaw/1
  Bus Selector5/1 -> yaw/1, Sum1/2  "<yaw>"
  yaw_ref/1 -> Sum1/1

== system flightController/Flight Control Systems/Flight Controller PID/gravity feedforward//equilibrium thrust ==
  note: ALTITUDE
  states_estim : Inport
  PosZ : Inport  Port=2
  takeoff_flag : Inport  Port=3
  Bus Selector6 : BusSelector  OutputSignals=Z,dz
  D_z : Gain  Gain=0.3  ParamDataTypeStr=single  OutDataTypeStr=single  SaturateOnIntegerOverflow=on
  P_z : Gain  Gain=0.8  ParamDataTypeStr=single  OutDataTypeStr=single  SaturateOnIntegerOverflow=on
  SaturationThrust : Saturate  UpperLimit=4*Controller.totalThrustMaxRelative*Controller.motorsThrustPerMotorMax  LowerLimit=-4*Controller.totalThrustMaxRelative*Controller.motorsThrustPerMotorMax  OutDataTypeStr=single
  Sum15 : Sum  Inputs=|+-  AccumDataTypeStr=single  OutDataTypeStr=single  SaturateOnIntegerOverflow=on
  Sum3 : Sum  Inputs=+-|  AccumDataTypeStr=single  OutDataTypeStr=single  SaturateOnIntegerOverflow=on
  Sum4 : Sum  Inputs=++|  AccumDataTypeStr=single  OutDataTypeStr=single  SaturateOnIntegerOverflow=on
  TakeoffOrControl_Switch : Switch  Criteria=u2 > Threshold
  takeoff_gain : Gain  Gain=Controller.takeoffGain  ParamDataTypeStr=single  OutDataTypeStr=single  SaturateOnIntegerOverflow=on
  w0 : Constant  Value=-g*Vehicle.Airframe.mass  OutDataTypeStr=single  SampleTime=Ts
  altitude_cmd : Outport  VectorParamsAs1DForOutWhenUnconnected=off
  wires:
  Sum3/1 -> P_z/1  "errZ"
  TakeoffOrControl_Switch/1 -> Sum4/2
  Bus Selector6/1 -> Sum3/2  "<Z>"
  Bus Selector6/2 -> D_z/1  "<dz>"
  w0/1 -> Sum4/1, takeoff_gain/1
  D_z/1 -> Sum15/2  "dz"
  takeoff_gain/1 -> TakeoffOrControl_Switch/1
  takeoff_flag/1 -> TakeoffOrControl_Switch/2
  PosZ/1 -> Sum3/1
  P_z/1 -> Sum15/1
  Sum15/1 -> TakeoffOrControl_Switch/3
  Sum4/1 -> SaturationThrust/1
  SaturationThrust/1 -> altitude_cmd/1
  states_estim/1 -> Bus Selector6/1

== system flightController/Flight Control Systems/Flight Controller PID/thrustsToMotorCommands ==
  thrusts_refin : Inport
  MotorDirections : Gain  Gain=[1 -1 1 -1]
  Saturation5 : Saturate  UpperLimit=Vehicle.Motor.maxLimit  LowerLimit=Vehicle.Motor.minLimit
  ThrustToMotorCommand : Gain  Gain=-Vehicle.Motor.thrustToMotorCommand
  "cmd1, cmd2, cmd3, cmd4" : Display
  "f1, f2, f3, f4" : Display
  motors_cmdout : Outport  VectorParamsAs1DForOutWhenUnconnected=off
  wires:
  Saturation5/1 -> MotorDirections/1
  MotorDirections/1 -> motors_cmdout/1, "cmd1, cmd2, cmd3, cmd4"/1
  ThrustToMotorCommand/1 -> Saturation5/1
  thrusts_refin/1 -> "f1, f2, f3, f4"/1, ThrustToMotorCommand/1

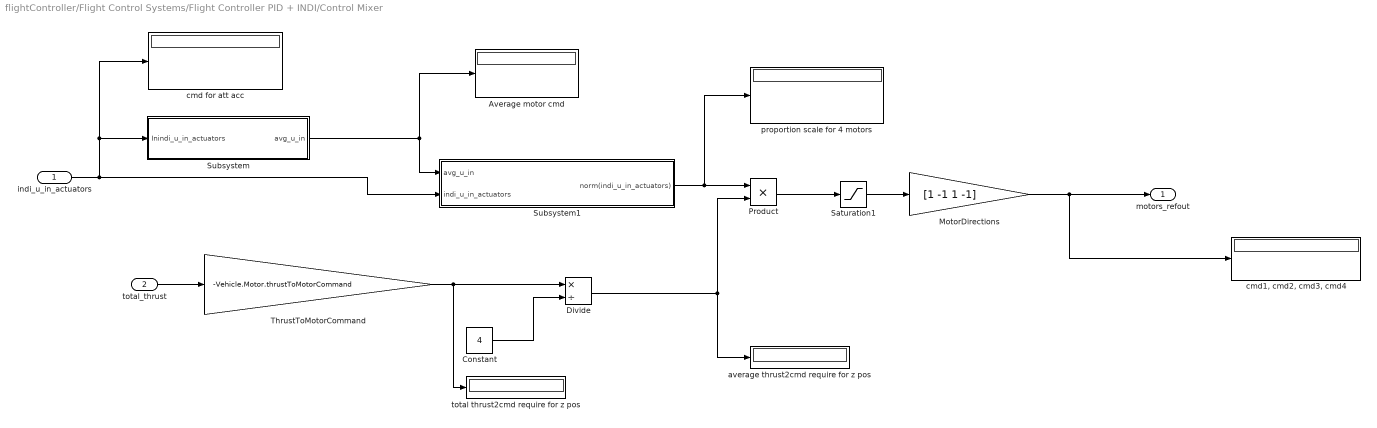
== system flightController/Flight Control Systems/Flight Controller PID + INDI/Control Mixer ==
  indi_u_in_actuators : Inport
  total_thrust : Inport  Port=2
  Average motor cmd : Display
  Constant : Constant  Value=4  OutDataTypeStr=single
  Divide : Product  Inputs=*/
  MotorDirections : Gain  Gain=[1 -1 1 -1]
  Product : Product
  Saturation1 : Saturate  UpperLimit=Vehicle.Motor.maxLimit  LowerLimit=Vehicle.Motor.minLimit
  Subsystem : Subsystem
  Subsystem1 : Subsystem
  ThrustToMotorCommand : Gain  Gain=-Vehicle.Motor.thrustToMotorCommand
  average thrust2cmd require for z pos : Display
  cmd for att acc : Display
  "cmd1, cmd2, cmd3, cmd4" : Display
  proportion scale for 4 motors : Display
  total thrust2cmd require for z pos : Display
  motors_refout : Outport
  wires:
  total_thrust/1 -> ThrustToMotorCommand/1
  ThrustToMotorCommand/1 -> total thrust2cmd require for z pos/1, Divide/1
  indi_u_in_actuators/1 -> Subsystem/1(Inindi_u_in_actuators), cmd for att acc/1, Subsystem1/2(indi_u_in_actuators)
  Subsystem/1(avg_u_in) -> Average motor cmd/1, Subsystem1/1(avg_u_in)
  Subsystem1/1(norm(indi_u_in_actuators)) -> Product/1, proportion scale for 4 motors/1
  Divide/1 -> average thrust2cmd require for z pos/1, Product/2
  Product/1 -> Saturation1/1
  Saturation1/1 -> MotorDirections/1
  MotorDirections/1 -> "cmd1, cmd2, cmd3, cmd4"/1, motors_refout/1
  Constant/1 -> Divide/2

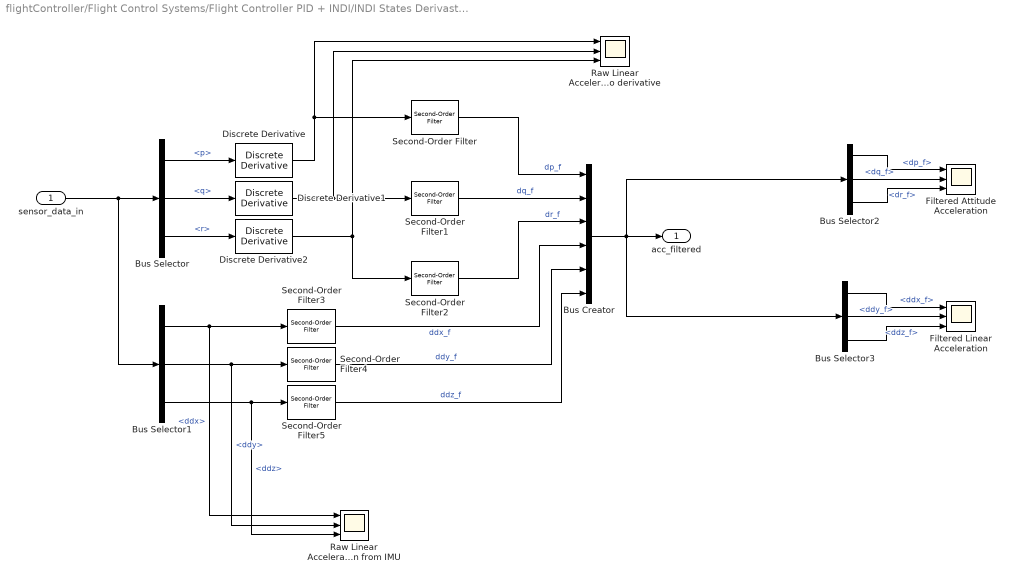
== system flightController/Flight Control Systems/Flight Controller PID + INDI/INDI States Derivastive Estimation ==
  sensor_data_in : Inport
  Bus Creator : BusCreator  Inputs=6
  Bus Selector : BusSelector  OutputSignals=p,q,r
  Bus Selector1 : BusSelector  OutputSignals=ddx,ddy,ddz
  Bus Selector2 : BusSelector  OutputSignals=dp_f,dq_f,dr_f
  Bus Selector3 : BusSelector  OutputSignals=ddx_f,ddy_f,ddz_f
  Discrete Derivative : simulink/Discrete/Discrete Derivative  gainval=1.0  ICPrevScaledInput=0.0  OutMin=[]  OutMax=[]  OutDataType=fixdt(1, 16)  OutScaling=2^-10  DoSatur=off
  Discrete Derivative1 : simulink/Discrete/Discrete Derivative  gainval=1.0  ICPrevScaledInput=0.0  OutMin=[]  OutMax=[]  OutDataType=fixdt(1, 16)  OutScaling=2^-10  DoSatur=off
  Discrete Derivative2 : simulink/Discrete/Discrete Derivative  gainval=1.0  ICPrevScaledInput=0.0  OutMin=[]  OutMax=[]  OutDataType=fixdt(1, 16)  OutScaling=2^-10  DoSatur=off
  Filtered Attitude Acceleration : Scope  NumInputPorts=3
  Filtered Linear Acceleration : Scope  NumInputPorts=3
  Raw Linear Acceleration from Gyro derivative : Scope  NumInputPorts=3
  Raw Linear Acceleration from IMU : Scope  NumInputPorts=3
  Second-Order Filter{,1..5} (6 alike) : spsSecondOrderFilterLib/Second-Order Filter  FilterType=Lowpass  Fo=7.9577  Zeta=0.55  Ts=0.005  Initialize=on  Vac_Init="[0,  0,  60]"  Vdc_Init=0  PlotResponse=off  FreqRange=[0, 500, 1]
      settings: SourceProductBaseCode=PS
  acc_filtered : Outport
  wires:
  sensor_data_in/1 -> Bus Selector/1, Bus Selector1/1
  Second-Order Filter/1 -> Bus Creator/1  "dp_f"
  Second-Order Filter1/1 -> Bus Creator/2  "dq_f"
  Second-Order Filter2/1 -> Bus Creator/3  "dr_f"
  Bus Selector/1 -> Discrete Derivative/1  "<p>"
  Bus Selector/2 -> Discrete Derivative1/1  "<q>"
  Bus Selector/3 -> Discrete Derivative2/1  "<r>"
  Discrete Derivative/1 -> Second-Order Filter/1, Raw Linear Acceleration from Gyro derivative/1
  Discrete Derivative1/1 -> Second-Order Filter1/1, Raw Linear Acceleration from Gyro derivative/2
  Discrete Derivative2/1 -> Second-Order Filter2/1, Raw Linear Acceleration from Gyro derivative/3
  Bus Selector1/1 -> Second-Order Filter3/1, Raw Linear Acceleration from IMU/1  "<ddx>"
  Bus Selector1/2 -> Second-Order Filter4/1, Raw Linear Acceleration from IMU/2  "<ddy>"
  Bus Selector1/3 -> Second-Order Filter5/1, Raw Linear Acceleration from IMU/3  "<ddz>"
  Second-Order Filter3/1 -> Bus Creator/4  "ddx_f"
  Second-Order Filter4/1 -> Bus Creator/5  "ddy_f"
  Second-Order Filter5/1 -> Bus Creator/6  "ddz_f"
  Bus Selector2/2 -> Filtered Attitude Acceleration/2  "<dq_f>"
  Bus Selector2/3 -> Filtered Attitude Acceleration/3  "<dr_f>"
  Bus Selector2/1 -> Filtered Attitude Acceleration/1  "<dp_f>"
  Bus Selector3/3 -> Filtered Linear Acceleration/3  "<ddz_f>"
  Bus Selector3/1 -> Filtered Linear Acceleration/1  "<ddx_f>"
  Bus Creator/1 -> Bus Selector3/1, Bus Selector2/1, acc_filtered/1
  Bus Selector3/2 -> Filtered Linear Acceleration/2  "<ddy_f>"

== system flightController/Flight Control Systems/Flight Controller PID + INDI/Inner INDI Loop ==
  att_acc_ref : Inport
  acc_filtered : Inport  Port=2
  Add : Sum
  Add1 : Sum
  Bus Selector1 : BusSelector  OutputSignals=dp_ref,dq_ref,dr_ref
  Bus Selector2 : BusSelector  OutputSignals=dp_f,dq_f,dr_f
  G2 : Gain  Gain=INDI.G2  Multiplication=Matrix(K*u)
  Mux : Mux  Inputs=3
  Mux1 : Mux  Inputs=3
  Plus : Sum  Inputs=|+-
  Unit Delay : UnitDelay  InitialCondition=[0 0 0 0]  SampleTime=-1  HasFrameUpgradeWarning=on
  Unit Delay1 : UnitDelay  SampleTime=-1  HasFrameUpgradeWarning=on
  inv(G1+G2) : Gain  Gain=INDI.G1G2_inv  Multiplication=Matrix(K*u)
  motor-speed to motor-cmd : Subsystem
  indi_u_in_actuators : Outport
  wires:
  Plus/1 -> Add/1  "attitude_acc_error"
  Add/1 -> inv(G1+G2)/1
  Unit Delay/1 -> G2/1
  G2/1 -> Add/2
  inv(G1+G2)/1 -> Add1/1, Unit Delay/1  "delta_motor_w"
  Unit Delay1/1 -> Add1/2  "motor_w_f"
  Add1/1 -> Unit Delay1/1, motor-speed to motor-cmd/1(motor_w_c)  "motor_w_c"
  motor-speed to motor-cmd/1(motors_refout) -> indi_u_in_actuators/1
  att_acc_ref/1 -> Bus Selector1/1
  Bus Selector1/1 -> Mux/1  "<dp_ref>"
  Bus Selector1/2 -> Mux/2  "<dq_ref>"
  Bus Selector1/3 -> Mux/3  "<dr_ref>"
  Mux/1 -> Plus/1
  Bus Selector2/3 -> Mux1/3  "<dr_f>"
  Bus Selector2/2 -> Mux1/2  "<dq_f>"
  Bus Selector2/1 -> Mux1/1  "<dp_f>"
  Mux1/1 -> Plus/2
  acc_filtered/1 -> Bus Selector2/1

== system flightController/Flight Control Systems/Flight Controller PID + INDI/PD Attitude Controller ==
  note: ATTITUDE
  refAttitude : Inport
  states_estim : Inport  Port=2
  Bus Creator : BusCreator  Inputs=3
  Bus Selector : BusSelector  OutputSignals=pitch,roll,yaw
  Bus Selector3 : BusSelector  OutputSignals=pitch,roll,yaw
  Bus Selector4 : BusSelector  OutputSignals=p,q,r
  D_pr : Gain  Gain=[0.002;0.0028;1]
  Demux1 : Demux  Outputs=3
  Mux : Mux  Inputs=3
  Mux1 : Mux  Inputs=3
  Mux2 : Mux  Inputs=3
  P_pr : Gain  Gain=[0.013;0.01;1]
  Sum1 : Sum  Inputs=|+-
  Sum19 : Sum  Inputs=+-|
  att_acc_ref : Outport
  wires:
  Sum19/1 -> P_pr/1  "roll/pitch/yaw error"
  states_estim/1 -> Bus Selector3/1, Bus Selector4/1
  P_pr/1 -> Sum1/1  "p/q/r ref"
  Mux1/1 -> Sum1/2
  Sum1/1 -> D_pr/1  "p/q/r error"
  Bus Selector4/2 -> Mux1/2  "<q>"
  Bus Selector4/1 -> Mux1/1  "<p>"
  Bus Selector4/3 -> Mux1/3  "<r>"
  D_pr/1 -> Demux1/1
  Demux1/1 -> Bus Creator/1  "dp_ref"
  Demux1/2 -> Bus Creator/2  "dq_ref"
  Demux1/3 -> Bus Creator/3  "dr_ref"
  Bus Creator/1 -> att_acc_ref/1
  refAttitude/1 -> Bus Selector/1
  Bus Selector/1 -> Mux/1  "<pitch>"
  Bus Selector/2 -> Mux/2  "<roll>"
  Bus Selector/3 -> Mux/3  "<yaw>"
  Bus Selector3/1 -> Mux2/1  "<pitch>"
  Bus Selector3/2 -> Mux2/2  "<roll>"
  Bus Selector3/3 -> Mux2/3  "<yaw>"
  Mux/1 -> Sum19/1
  Mux2/1 -> Sum19/2

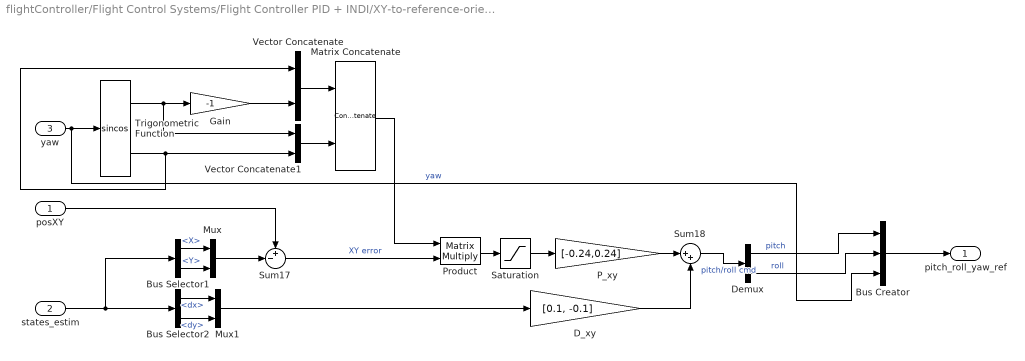
== system flightController/Flight Control Systems/Flight Controller PID + INDI/XY-to-reference-orientation ==
  posXY : Inport
  states_estim : Inport  Port=2
  yaw : Inport  Port=3
  Bus Creator : BusCreator  Inputs=3
  Bus Selector1 : BusSelector  OutputSignals=X,Y
  Bus Selector2 : BusSelector  OutputSignals=dx,dy
  D_xy : Gain  Gain=[0.1, -0.1]  ParamDataTypeStr=single  OutDataTypeStr=single  SaturateOnIntegerOverflow=on
  Demux : Demux  Outputs=2
  Gain : Gain  Gain=-1
  Matrix Concatenate : Concatenate  Mode=Multidimensional array  ConcatenateDimension=2
  Mux : Mux  Inputs=2
  Mux1 : Mux  Inputs=2
  P_xy : Gain  Gain=[-0.24,0.24]  ParamDataTypeStr=single  OutDataTypeStr=single  SaturateOnIntegerOverflow=on
  Product : Product  Multiplication=Matrix(*)  OutDataTypeStr=single  RndMeth=Zero
  Saturation : Saturate  UpperLimit=3  LowerLimit=-3  OutDataTypeStr=single
  Sum17 : Sum  Inputs=+-|  AccumDataTypeStr=single
  Sum18 : Sum  Inputs=|++  AccumDataTypeStr=single  OutDataTypeStr=single  SaturateOnIntegerOverflow=on
  Trigonometric Function : Trigonometry  Operator=sincos
  Vector Concatenate : Concatenate
  Vector Concatenate1 : Concatenate
  pitch_roll_yaw_ref : Outport  VectorParamsAs1DForOutWhenUnconnected=off
  wires:
  yaw/1 -> Bus Creator/3, Trigonometric Function/1  "yaw"
  Saturation/1 -> P_xy/1
  P_xy/1 -> Sum18/1
  Sum17/1 -> Product/2  "XY error"
  posXY/1 -> Sum17/1
  Bus Selector2/1 -> Mux1/1  "<dx>"
  states_estim/1 -> Bus Selector1/1, Bus Selector2/1
  D_xy/1 -> Sum18/2
  Bus Selector1/1 -> Mux/1  "<X>"
  Product/1 -> Saturation/1
  Trigonometric Function/1 -> Gain/1, Vector Concatenate1/1
  Trigonometric Function/2 -> Vector Concatenate1/2, Vector Concatenate/1
  Gain/1 -> Vector Concatenate/2
  Vector Concatenate/1 -> Matrix Concatenate/1
  Vector Concatenate1/1 -> Matrix Concatenate/2
  Matrix Concatenate/1 -> Product/1
  Bus Selector1/2 -> Mux/2  "<Y>"
  Mux/1 -> Sum17/2
  Mux1/1 -> D_xy/1
  Bus Selector2/2 -> Mux1/2  "<dy>"
  Sum18/1 -> Demux/1  "pitch/roll cmd"
  Bus Creator/1 -> pitch_roll_yaw_ref/1
  Demux/1 -> Bus Creator/1  "pitch"
  Demux/2 -> Bus Creator/2  "roll"

== system flightController/Flight Control Systems/Flight Controller PID + INDI/gravity feedforward//equilibrium thrust ==
  note: ALTITUDE
  states_estim : Inport
  PosZ : Inport  Port=2
  takeoff_flag : Inport  Port=3
  Bus Selector6 : BusSelector  OutputSignals=Z,dz
  D_z : Gain  Gain=0.3  ParamDataTypeStr=single  OutDataTypeStr=single  SaturateOnIntegerOverflow=on
  P_z : Gain  Gain=0.8  ParamDataTypeStr=single  OutDataTypeStr=single  SaturateOnIntegerOverflow=on
  SaturationThrust : Saturate  UpperLimit=4*Controller.totalThrustMaxRelative*Controller.motorsThrustPerMotorMax  LowerLimit=-4*Controller.totalThrustMaxRelative*Controller.motorsThrustPerMotorMax  OutDataTypeStr=single
  Sum15 : Sum  Inputs=|+-  AccumDataTypeStr=single  OutDataTypeStr=single  SaturateOnIntegerOverflow=on
  Sum3 : Sum  Inputs=+-|  AccumDataTypeStr=single  OutDataTypeStr=single  SaturateOnIntegerOverflow=on
  Sum4 : Sum  Inputs=++|  AccumDataTypeStr=single  OutDataTypeStr=single  SaturateOnIntegerOverflow=on
  TakeoffOrControl_Switch : Switch  Criteria=u2 > Threshold
  takeoff_gain : Gain  Gain=Controller.takeoffGain  ParamDataTypeStr=single  OutDataTypeStr=single  SaturateOnIntegerOverflow=on
  w0 : Constant  Value=-g*Vehicle.Airframe.mass  OutDataTypeStr=single  SampleTime=Ts
  altitude_cmd : Outport  VectorParamsAs1DForOutWhenUnconnected=off
  wires:
  Sum3/1 -> P_z/1  "errZ"
  TakeoffOrControl_Switch/1 -> Sum4/2
  Bus Selector6/1 -> Sum3/2  "<Z>"
  Bus Selector6/2 -> D_z/1  "<dz>"
  w0/1 -> Sum4/1, takeoff_gain/1
  D_z/1 -> Sum15/2  "dz"
  takeoff_gain/1 -> TakeoffOrControl_Switch/1
  takeoff_flag/1 -> TakeoffOrControl_Switch/2
  PosZ/1 -> Sum3/1
  P_z/1 -> Sum15/1
  Sum15/1 -> TakeoffOrControl_Switch/3
  Sum4/1 -> SaturationThrust/1
  SaturationThrust/1 -> altitude_cmd/1
  states_estim/1 -> Bus Selector6/1

== system flightController/Flight Control Systems/Flight Controller INDI/Inner INDI Loop/motor-speed to motor-cmd ==
  motor_w_c : Inport
  Motor directions : Gain  Gain=[1 -1 1 -1]  ParamDataTypeStr=single  OutDataTypeStr=Inherit: Inherit via back propagation  SaturateOnIntegerOverflow=on
  Saturation5 : Saturate  UpperLimit=Vehicle.Motor.maxLimit  LowerLimit=Vehicle.Motor.minLimit  OutDataTypeStr=Inherit: Inherit via back propagation
  Square : Math  Operator=square  SaturateOnIntegerOverflow=on
  speed-to-command : Gain  Gain=1/Vehicle.Motor.commandToW2Gain
  motors_refout : Outport
  wires:
  motor_w_c/1 -> Square/1
  Square/1 -> speed-to-command/1
  Saturation5/1 -> Motor directions/1
  speed-to-command/1 -> Saturation5/1
  Motor directions/1 -> motors_refout/1

== system flightController/Flight Control Systems/Flight Controller PID + INDI/Control Mixer/Subsystem ==
  Inindi_u_in_actuators : Inport
  CancelMotorDirections : Gain  Gain=[1 -1 1 -1]
  Constant : Constant  Value=4  OutDataTypeStr=single
  Demux : Demux
  Display : Display
  Divide : Product  Inputs=*/
  Sum : Sum  Inputs=++++
  avg_u_in : Outport
  wires:
  Demux/4 -> Sum/4
  Constant/1 -> Divide/2
  Demux/2 -> Sum/2
  Demux/1 -> Sum/1
  Divide/1 -> avg_u_in/1
  Sum/1 -> Divide/1
  Demux/3 -> Sum/3
  Inindi_u_in_actuators/1 -> Display/1, CancelMotorDirections/1
  CancelMotorDirections/1 -> Demux/1

== system flightController/Flight Control Systems/Flight Controller PID + INDI/Control Mixer/Subsystem1 ==
  avg_u_in : Inport
  indi_u_in_actuators : Inport  Port=2
  CancelMotorDirections : Gain  Gain=[1 -1 1 -1]
  Demux : Demux
  Divide{,1..3} (4 alike) : Product  Inputs=*/
  Mux : Mux
  norm(indi_u_in_actuators) : Outport
  wires:
  Divide1/1 -> Mux/2  "norm(indi_u_in_actuators[1])"
  avg_u_in/1 -> Divide1/2, Divide3/2, Divide2/2, Divide/2
  Demux/4 -> Divide3/1
  Demux/1 -> Divide/1
  Demux/3 -> Divide2/1
  Demux/2 -> Divide1/1
  CancelMotorDirections/1 -> Demux/1
  Divide2/1 -> Mux/3  "norm(indi_u_in_actuators[2])"
  Mux/1 -> norm(indi_u_in_actuators)/1
  Divide3/1 -> Mux/4  "norm(indi_u_in_actuators[3])"
  Divide/1 -> Mux/1  "norm(indi_u_in_actuators[0])"
  indi_u_in_actuators/1 -> CancelMotorDirections/1

== system flightController/Flight Control Systems/Flight Controller PID + INDI/Inner INDI Loop/motor-speed to motor-cmd ==
  motor_w_c : Inport
  Motor directions : Gain  Gain=[1 -1 1 -1]  ParamDataTypeStr=single  OutDataTypeStr=Inherit: Inherit via back propagation  SaturateOnIntegerOverflow=on
  Saturation5 : Saturate  UpperLimit=Vehicle.Motor.maxLimit  LowerLimit=Vehicle.Motor.minLimit  OutDataTypeStr=Inherit: Inherit via back propagation
  Square : Math  Operator=square  SaturateOnIntegerOverflow=on
  speed-to-command : Gain  Gain=1/Vehicle.Motor.commandToW2Gain
  motors_refout : Outport
  wires:
  motor_w_c/1 -> Square/1
  Square/1 -> speed-to-command/1
  Saturation5/1 -> Motor directions/1
  speed-to-command/1 -> Saturation5/1
  Motor directions/1 -> motors_refout/1
